simulink model "first_model"  (R2025a)
settings: Solver=ode23t  StartTime=0.0  StopTime=4  MaxStep=1e-5  RelTol=1e-3
libraries: spsDiodeLib x7, spsDCMachineLib x2, spsDCVoltageSourceLib x2, simulink x2, spsSeriesRLCBranchLib x2, spsBreakerLib x1, spsGroundLib x1, spsIGBTDiodeLib x1, spsThreePhaseProgrammableVoltageSourceLib x1, spsVoltageMeasurementLib x1, sps_lib x1
settings Model: Creator=Yunus Tosun  LastModifiedBy=Yunus Tosun
settings SolverCC: ZeroCrossAlgorithm=Adaptive

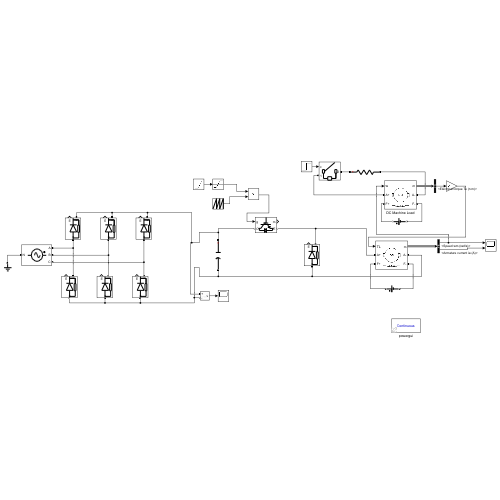
[thumbnail: Simulink's stored preview of the top-level diagram]
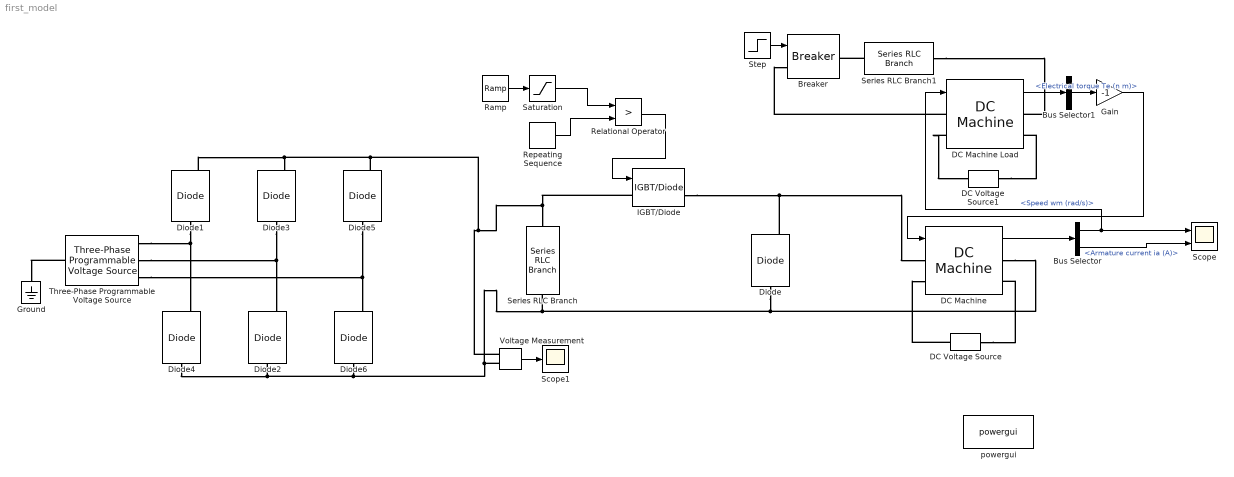
== system first_model ==
  Breaker : spsBreakerLib/Breaker  InitialState=0  SwitchingTimes="[1/60  5/60]"  External=on  BreakerResistance=0.01  SnubberResistance=1e6  SnubberCapacitance=inf  Measurements=None  MoreParameters=on  NoBreakLoop=off
  Bus Selector : BusSelector  OutputSignals=Speed wm (rad/s),Armature current ia (A)
  Bus Selector1 : BusSelector  OutputSignals=Electrical torque Te (n m)
  DC Machine : spsDCMachineLib/DC Machine  PresetModel=No  MechanicalLoad=Torque TL  FieldType=Wound  ShowDetailedParameters=on  MeasurementBus=off  RLa="[ 1.07  0.0245]"  RLf="[ 210  23]"  Laf=1.18  MachineConstant=Torque constant (N.m/A)  Ke=1.8  Kt=1.8  J=0.06  Bm=0.0032  Tf=0.3  w0=0  Ifinit=1.04761904756944  TsPowergui=0  TsBlock=-1
  DC Machine Load : spsDCMachineLib/DC Machine  PresetModel=No  MechanicalLoad=Speed w  FieldType=Wound  ShowDetailedParameters=on  MeasurementBus=off  RLa="[ 1.07  0.0245]"  RLf="[ 210  23]"  Laf=1.18  MachineConstant=Torque constant (N.m/A)  Ke=1.8  Kt=1.8  J=0.06  Bm=0.0032  Tf=0.3  w0=0  Ifinit=1.04761904761905  TsPowergui=0  TsBlock=-1
  DC Voltage Source : spsDCVoltageSourceLib/DC Voltage Source  Amplitude=220  Measurements=None
  DC Voltage Source1 : spsDCVoltageSourceLib/DC Voltage Source  Amplitude=220  Measurements=None
  Diode{,1..6} (7 alike) : spsDiodeLib/Diode  Ron=0.001  Lon=0  Vf=0.8  IC=0  UseSnubber=0  Rs=500  Cs=250e-9  Measurements=on
  Gain : Gain  Gain=-1
  Ground : spsGroundLib/Ground  LConnTagsString=a
  IGBT/Diode : spsIGBTDiodeLib/IGBT//Diode  Ron=1e-3  Rs=1e5  Cs=inf  Measurements=on
  Ramp : simulink/Sources/Ramp  slope=0.425  start=0  InitialOutput=0
  Relational Operator : RelationalOperator  Operator=>  OutDataTypeStr=boolean  RndMeth=Simplest  InputSameDT=off
  Repeating Sequence : simulink/Sources/Repeating Sequence  rep_seq_t=[0 0.0001]  rep_seq_y=[0 1]
  Saturation : Saturate  UpperLimit=0.85  LowerLimit=0
  Scope : Scope  NumInputPorts=2
      settings: ActiveDisplayYMinimum=-23.528143646666418  ActiveDisplayYMaximum=148.9323473339966
  Scope1 : Scope
      settings: ActiveDisplayYMinimum=139.47565629905122  ActiveDisplayYMaximum=264.4727330125051
  Series RLC Branch : spsSeriesRLCBranchLib/Series RLC Branch  LConnTagsString=__new0  RConnTagsString=__new0  BranchType=C  Resistance=1  Inductance=1e-3  SetiL0=off  InitialCurrent=0  Capacitance=1000e-6  Setx0=off  InitialVoltage=0  Measurements=None
  Series RLC Branch1 : spsSeriesRLCBranchLib/Series RLC Branch  LConnTagsString=__new0  RConnTagsString=__new0  BranchType=R  Resistance=12  Inductance=1e-3  SetiL0=off  InitialCurrent=0  Capacitance=1e-6  Setx0=off  InitialVoltage=0  Measurements=None
  Step : Step  Time=2.5  SampleTime=0
  Three-Phase Programmable Voltage Source : spsThreePhaseProgrammableVoltageSourceLib/Three-Phase Programmable Voltage Source  PositiveSequence="[150  0 50]"  VariationEntity=None  VariationType=Table of time-amplitude pairs  VariationTypeAlt=Step  VariationStep=0.5  VariationRate=10  VariationMagnitude=0.3  VariationFrequency=2  VariationTiming=[1 2]  VariationPhaseA=off  Amplitudes=[1 0.8 1.2 1.0]  TimeValues=[0 0.1 0.15 0.2]  HarmonicGeneration=off  HarmonicA=[3 0.2 -25 0]  HarmonicB=[2 0.15 35 2]  Timing="[0.05  3]"  BusType=swing  Pref=0  Qref=0  Qmin=-inf  Qmax=inf
  Voltage Measurement : spsVoltageMeasurementLib/Voltage Measurement  PhasorSimulation=off  OutputType=Complex  PSBequivalent=0
  powergui : sps_lib/powergui  Priority=1  SimulationMode=Continuous  SampleTime=50e-6  frequency=60  Iterations=50  frequencyindice=0  Pbase=100e6  ErrMax=1e-4  UnitsV=kV  UnitsW=MW  buscounter=0  FunctionMessages=off  echomessages=off  EnableUseOfTLC=off  CurrentSourceSwitches=off  DisableSnubberDevices=off  DisableRonSwitches=off  DisableVfSwitches=off  DisplayEquations=off  AutomaticDiscreteSolvers=off  SolverType=Tustin/Backward Euler (TBE)  Interpol=off  ExternalGateDelay=off  methode=off  Ts=100  x0status=blocks  SPID=on  SwTol=0  HookPort=off  NonlinearTolerance=1e-4  nMaxIteration=100  ContinueOnMaxIteration=off  RestoreLinks=warning  ResistiveCurrentMeasurement=off  Frange=[0:2:500]  Ylog=off  Xlog=on  ShowGrid=off  save=off  variable=ZData  structure=0  ZoomFFT=off  StartTime=0.0  cycles=1  DisplayStyle=1  fundamental=60  FreqAxis=off  MaxFrequency=1000  frequencyindicesteady=1  RmsSteady=1  display=off
  wires:
  DC Machine/1 -> Bus Selector/1
  Bus Selector/2 -> Scope/2  "<Armature current ia (A)>"
  Bus Selector/1 -> DC Machine Load/1, Scope/1  "<Speed wm (rad/s)>"
  Voltage Measurement/1 -> Scope1/1
  Ramp/1 -> Saturation/1
  Saturation/1 -> Relational Operator/1
  Repeating Sequence/1 -> Relational Operator/2
  Relational Operator/1 -> IGBT/Diode/1
  DC Machine Load/1 -> Bus Selector1/1
  Bus Selector1/1 -> Gain/1  "<Electrical torque Te (n m)>"
  Gain/1 -> DC Machine/1
  Step/1 -> Breaker/1
  connections:
  DC Voltage Source/LConn1 -- DC Machine/RConn2
  DC Voltage Source/RConn1 -- DC Machine/LConn2
  IGBT/Diode/RConn1 -- Diode/RConn1 -- DC Machine/LConn1
  Three-Phase Programmable Voltage Source/LConn1 -- Ground/LConn1
  Diode1/LConn1 -- Three-Phase Programmable Voltage Source/RConn1 -- Diode4/RConn1
  Diode3/LConn1 -- Three-Phase Programmable Voltage Source/RConn2 -- Diode2/RConn1
  Diode5/LConn1 -- Three-Phase Programmable Voltage Source/RConn3 -- Diode6/RConn1
  Diode3/RConn1 -- Diode1/RConn1 -- Diode5/RConn1 -- Voltage Measurement/LConn1 -- Series RLC Branch/LConn1 -- IGBT/Diode/LConn1
  Voltage Measurement/LConn2 -- DC Machine/RConn1 -- Diode/LConn1 -- Series RLC Branch/RConn1 -- Diode2/LConn1 -- Diode4/LConn1 -- Diode6/LConn1
  DC Machine Load/LConn2 -- DC Voltage Source1/RConn1
  DC Voltage Source1/LConn1 -- DC Machine Load/RConn2
  Series RLC Branch1/LConn1 -- Breaker/RConn1
  DC Machine Load/LConn1 -- Breaker/LConn1
  Series RLC Branch1/RConn1 -- DC Machine Load/RConn1
